simulink library "Reinterpolation"  (R2016b)
settings: Solver=VariableStepAuto  StartTime=0.0  StopTime=10.0  RelTol=1e-3
undefined symbols (not defined in the file): t_coords_reinterp
libraries: simulink x1
settings Model: Creator=cava_da  LastModifiedBy=cava_da
settings DataIOCC: ReturnWorkspaceOutputs=on
settings SFSimCC: SimUseLocalCustomCode=on
settings RTWCC: RTWUseLocalCustomCode=on

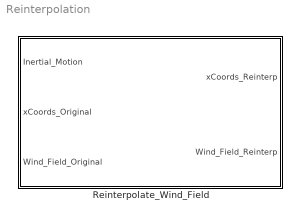
== system Reinterpolation ==
  Reinterpolate_Wind_Field : Subsystem  mask(Wind Field Reinterpolation){t_coords_reinterp=t_coords_reinterp}
      mask prompts: t_coords_reinterp "Relative time coordinates for reinterpolation"
      mask help:
      | This block reinterpolates the wind field using a vector of relative time coordinates.
      | These time coordinates specify a time difference with respect to the aircraft reference position used by the wind reconstruction algorithm (provided in Inertial_Motion).
      | To avoid sharp discontinuities in case the reinterpolation coordinates exceed the bounds of the original wind field, the original wind field is first artificially extended.

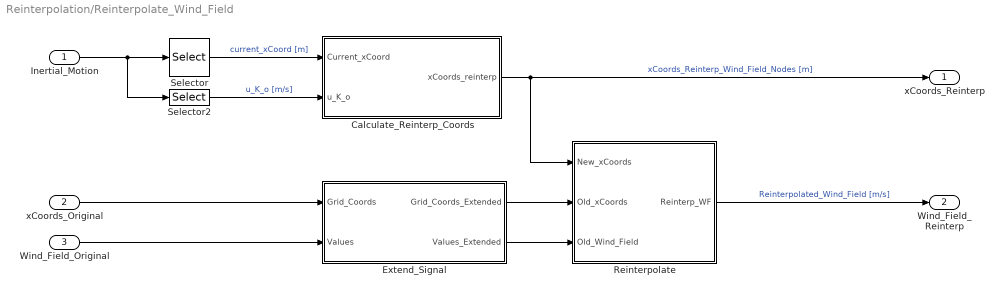
== system Reinterpolation/Reinterpolate_Wind_Field ==
  Inertial_Motion : Inport
  xCoords_Original : Inport  Port=2
  Wind_Field_Original : Inport  Port=3
  Calculate_Reinterp_Coords : Subsystem
  Extend_Signal : Subsystem  mask(Extend vector signal){N_nodes_ahead=50, N_nodes_behind=50}
      mask prompts: N_nodes_ahead "Nodes added ahead"; N_nodes_behind "Nodes added behind"
      mask help: Artificially extends a vector signal (such as an estimated wind field) by adding nodes ahead and behind. The values assigned to these nodes exponentially approach the time-averaged mean of the signal.
  Reinterpolate : Subsystem
  Selector : Selector  IndexOptions=Index vector (dialog)  Indices=1  OutputSizes=1
  Selector2 : Selector  IndexOptions=Index vector (dialog)  Indices=7  OutputSizes=1
  xCoords_Reinterp : Outport
  Wind_Field_Reinterp : Outport  Port=2
  wires:
  Reinterpolate/1(Reinterp_WF) -> Wind_Field_Reinterp/1  "Reinterpolated_Wind_Field [m/s]"
  Extend_Signal/1(Grid_Coords_Extended) -> Reinterpolate/2(Old_xCoords)
  Calculate_Reinterp_Coords/1(xCoords_reinterp) -> xCoords_Reinterp/1, Reinterpolate/1(New_xCoords)  "xCoords_Reinterp_Wind_Field_Nodes [m]"
  Selector2/1 -> Calculate_Reinterp_Coords/2(u_K_o)  "u_K_o [m/s]"
  Selector/1 -> Calculate_Reinterp_Coords/1(Current_xCoord)  "current_xCoord [m]"
  Wind_Field_Original/1 -> Extend_Signal/2(Values)
  Extend_Signal/2(Values_Extended) -> Reinterpolate/3(Old_Wind_Field)
  xCoords_Original/1 -> Extend_Signal/1(Grid_Coords)
  Inertial_Motion/1 -> Selector2/1, Selector/1

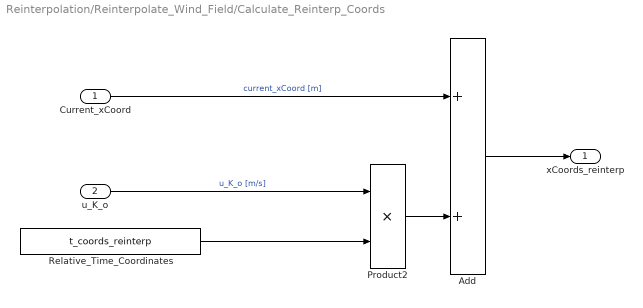
== system Reinterpolation/Reinterpolate_Wind_Field/Calculate_Reinterp_Coords ==
  Current_xCoord : Inport
  u_K_o : Inport  Port=2
  Add : Sum
  Product2 : Product  RndMeth=Zero
  Relative_Time_Coordinates : Constant  Value=t_coords_reinterp
  xCoords_reinterp : Outport
  wires:
  Current_xCoord/1 -> Add/1  "current_xCoord [m]"
  Product2/1 -> Add/2
  Add/1 -> xCoords_reinterp/1
  u_K_o/1 -> Product2/1  "u_K_o [m/s]"
  Relative_Time_Coordinates/1 -> Product2/2

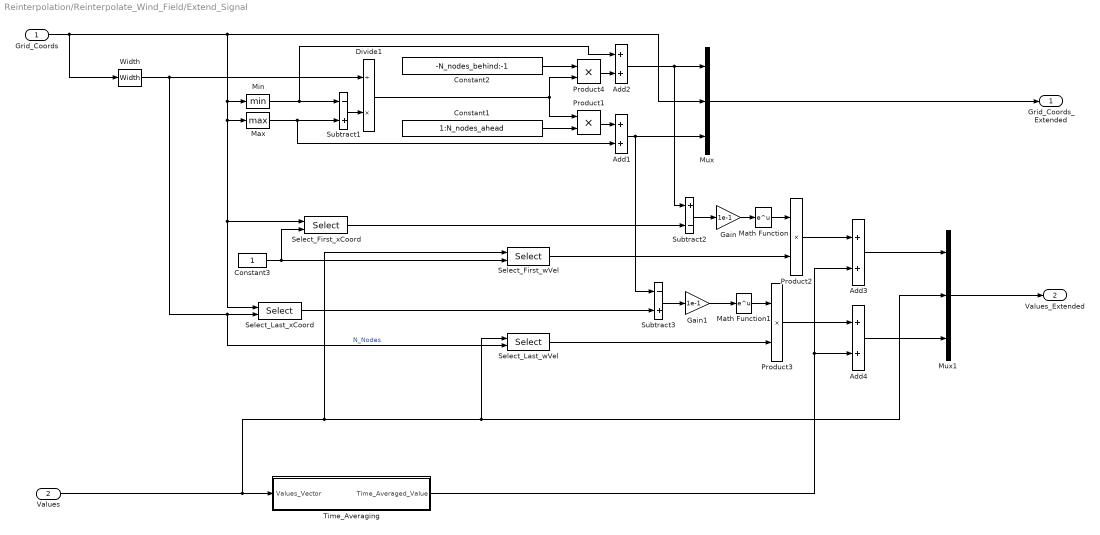
== system Reinterpolation/Reinterpolate_Wind_Field/Extend_Signal ==
  Grid_Coords : Inport
  Values : Inport  Port=2
  Add{1..4} (4 alike) : Sum
  Constant1 : Constant  Value=1:N_nodes_ahead
  Constant2 : Constant  Value=-N_nodes_behind:-1
  Constant3 : Constant
  Divide1 : Product  Inputs=/*
  Gain : Gain  Gain=1e-1
  Gain1 : Gain  Gain=1e-1
  Math Function : Math  SaturateOnIntegerOverflow=on
  Math Function1 : Math  SaturateOnIntegerOverflow=on
  Max : MinMax  Function=max
  Min : MinMax
  Mux : Mux  Inputs=3
  Mux1 : Mux  Inputs=3
  Product{1..4} (4 alike) : Product  RndMeth=Zero
  Select_First_wVel : Selector  IndexOptions=Index vector (port)  Indices=1  OutputSizes=1
  Select_First_xCoord : Selector  IndexOptions=Index vector (port)  Indices=1  OutputSizes=1
  Select_Last_wVel : Selector  IndexOptions=Index vector (port)  Indices=1  OutputSizes=1
  Select_Last_xCoord : Selector  IndexOptions=Index vector (port)  Indices=1  OutputSizes=1
  Subtract1 : Sum  Inputs=-+
  Subtract2 : Sum  Inputs=+-
  Subtract3 : Sum  Inputs=-+
  Time_Averaging : Subsystem
  Width : Width
  Grid_Coords_Extended : Outport
  Values_Extended : Outport  Port=2
  wires:
  Grid_Coords/1 -> Mux/2, Max/1, Select_First_xCoord/1, Select_Last_xCoord/1, Min/1, Width/1
  Time_Averaging/1(Time_Averaged_Value) -> Add3/2, Add4/2
  Values/1 -> Select_First_wVel/1, Mux1/2, Select_Last_wVel/1, Time_Averaging/1(Values_Vector)
  Max/1 -> Subtract1/2, Add1/2
  Subtract1/1 -> Divide1/2
  Constant1/1 -> Product1/2
  Divide1/1 -> Product1/1, Product4/2
  Product1/1 -> Add1/1
  Min/1 -> Subtract1/1, Add2/1
  Product4/1 -> Add2/2
  Constant2/1 -> Product4/1
  Add1/1 -> Mux/3, Subtract3/1
  Add2/1 -> Mux/1, Subtract2/1
  Mux/1 -> Grid_Coords_Extended/1
  Subtract2/1 -> Gain/1
  Math Function/1 -> Product2/1
  Select_First_wVel/1 -> Product2/2
  Product2/1 -> Add3/1
  Gain/1 -> Math Function/1
  Constant3/1 -> Select_First_wVel/2, Select_First_xCoord/2
  Select_First_xCoord/1 -> Subtract2/2
  Select_Last_xCoord/1 -> Subtract3/2
  Product3/1 -> Add4/1
  Math Function1/1 -> Product3/1
  Subtract3/1 -> Gain1/1
  Gain1/1 -> Math Function1/1
  Select_Last_wVel/1 -> Product3/2
  Add3/1 -> Mux1/1
  Add4/1 -> Mux1/3
  Mux1/1 -> Values_Extended/1
  Width/1 -> Select_Last_xCoord/2, Select_Last_wVel/2, Divide1/1  "N_Nodes"

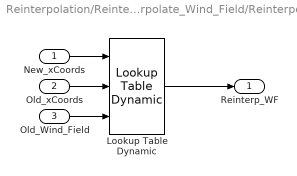
== system Reinterpolation/Reinterpolate_Wind_Field/Reinterpolate ==
  New_xCoords : Inport
  Old_xCoords : Inport  Port=2
  Old_Wind_Field : Inport  Port=3
  Lookup Table Dynamic : simulink/Lookup Tables/Lookup Table Dynamic  LookUpMeth=Interpolation-Use End Values  OutDataType=float('double')  OutScaling=[]  OutputDataTypeScalingMode=Specify via dialog  OutDataTypeStr=float('double')  DoSatur=off
  Reinterp_WF : Outport
  wires:
  Old_xCoords/1 -> Lookup Table Dynamic/2
  Old_Wind_Field/1 -> Lookup Table Dynamic/3
  Lookup Table Dynamic/1 -> Reinterp_WF/1
  New_xCoords/1 -> Lookup Table Dynamic/1

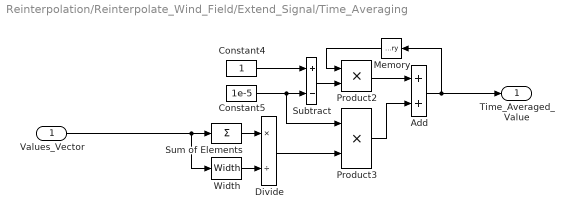
== system Reinterpolation/Reinterpolate_Wind_Field/Extend_Signal/Time_Averaging ==
  Values_Vector : Inport
  Add : Sum
  Constant4 : Constant
  Constant5 : Constant  Value=1e-5
  Divide : Product  Inputs=*/
  Memory : Memory
  Product2 : Product  RndMeth=Zero
  Product3 : Product  RndMeth=Zero
  Subtract : Sum  Inputs=+-
  Sum of Elements : Sum  Inputs=+
  Width : Width
  Time_Averaged_Value : Outport
  wires:
  Sum of Elements/1 -> Divide/1
  Width/1 -> Divide/2
  Constant4/1 -> Subtract/1
  Constant5/1 -> Subtract/2, Product3/1
  Add/1 -> Memory/1, Time_Averaged_Value/1
  Product2/1 -> Add/1
  Subtract/1 -> Product2/2
  Memory/1 -> Product2/1
  Product3/1 -> Add/2
  Divide/1 -> Product3/2
  Values_Vector/1 -> Sum of Elements/1, Width/1
